simulink model "Analog_Solution"  (R2017a)
settings: Solver=FixedStepDiscrete  StartTime=0.0  StopTime=inf  FixedStep=Ts_main  RelTol=1e-3  EnableMultiTasking=on
InitFcn:
  | clc
  | eval('ContrPrm_v1_1')
model workspace (MAT data in the model file):
  JoyW_sat = 10
values from neighbouring files (symbols this model uses):
  Afilt_Winch = (Amatr_Winch-L_Winch*Cmatr_Winch)    [ContrPrm_v1_1.m]
  AOsat = 10    [ContrPrm_v1_1.m]
  Bfilt_Winch = [L_Winch Bmatr_Winch]    [ContrPrm_v1_1.m]
  Cfilt_Winch = eye(2)    [ContrPrm_v1_1.m]
  Dfilt_Winch = zeros(2)    [ContrPrm_v1_1.m]
  JoyS_gain = 5    [ContrPrm_v1_1.m]
  JoyS_ofst = -2.5    [ContrPrm_v1_1.m]
  JoyS_sat = 9.2    [ContrPrm_v1_1.m]
  JoyW_gain = -5    [ContrPrm_v1_1.m]
  JoyW_ofst = -2.5    [ContrPrm_v1_1.m]
  KspdWinch = 1    [ContrPrm_v1_1.m]
  NPotSpdEst = 3    [ContrPrm_v1_1.m]
  Pot_gain = PotMax/5    (= 0.08)    [ContrPrm_v1_1.m]
  Pot_max = PotMax    (= 0.4)    [ContrPrm_v1_1.m]
  Pot_min = 0    [ContrPrm_v1_1.m]
  Pot_ofst = -0.0558    [ContrPrm_v1_1.m]
  Ts_1ms = 1e-3    (= 0.001)    [ContrPrm_v1_1.m]
  Ts_1s = 1    [ContrPrm_v1_1.m]
  WinchDrumRad = 0.1    [ContrPrm_v1_1.m]
  WinchMotPosAIgain = WinchRevMax/WinchVoltMax*rev2rad    (= 76)    [ContrPrm_v1_1.m]
  WinchMotTorqueMax = 13    [ContrPrm_v1_1.m]
  WinchRefSpdSup = 15/WinchDrumRad    (= 150)    [ContrPrm_v1_1.m]
  WinchTravelMin_m = -2    [ContrPrm_v1_1.m]
  WinchVoltMax = 10    [ContrPrm_v1_1.m]
  x0_Winch = [0;0]    [ContrPrm_v1_1.m]
undefined symbols (not defined in the file or in its folder): datevec, JoyFiltDen, JoyFiltNum, PotPosFiltDen, PotPosFiltNum, WinchPosFiltDen, WinchPosFiltNum, WinchSpdEstFiltDen, WinchSpdEstFiltNum
libraries: slrtlib x10, xpcnilib x6, simulink x6, xpcseriallib x4, xpcwalltimelib x1
(part 2 of 3)

== system Analog_Solution/Startup/Initialize Spooling Position/FirstDirectionDone? ==
  SpoolingGrenze1 : Inport
  Constant1 : Constant
  Constant2 : Constant  Value=0
  Delay : Delay  DelayLength=1  InitialCondition=0
  Relational Operator : RelationalOperator  Operator=<=  OutDataTypeStr=boolean  RndMeth=Simplest
  Sum : Sum  Inputs=|++
  Switch1 : Switch  Criteria=u2 > Threshold
  Switch2 : Switch  Criteria=u2 > Threshold
  FirstDirectionDone : Outport
  wires:
  Switch1/1 -> Sum/1
  Delay/1 -> Sum/2
  SpoolingGrenze1/1 -> Switch1/2
  Constant2/1 -> Switch2/3, Switch1/3
  Sum/1 -> Delay/1, Relational Operator/2
  Constant1/1 -> Switch2/1, Relational Operator/1, Switch1/1
  Relational Operator/1 -> Switch2/2
  Switch2/1 -> FirstDirectionDone/1

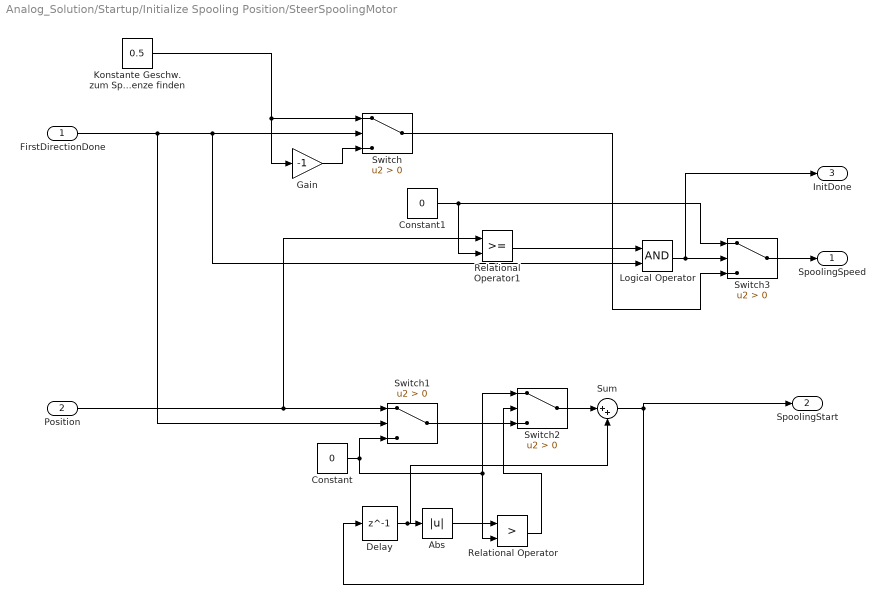
== system Analog_Solution/Startup/Initialize Spooling Position/SteerSpoolingMotor ==
  FirstDirectionDone : Inport
  Position : Inport  Port=2
  Abs : Abs
  Constant : Constant  Value=0
  Constant1 : Constant  Value=0
  Delay : Delay  DelayLength=1  InitialCondition=0
  Gain : Gain  Gain=-1
  Konstante Geschw. zum Spooling Grenze finden : Constant  Value=0.5
  Logical Operator : Logic  AllPortsSameDT=off  OutDataTypeStr=boolean
  Relational Operator : RelationalOperator  Operator=>  OutDataTypeStr=boolean  RndMeth=Simplest
  Relational Operator1 : RelationalOperator  OutDataTypeStr=boolean  RndMeth=Simplest
  Sum : Sum  Inputs=|++
  Switch{,1..3} (4 alike) : Switch  Criteria=u2 > Threshold
  SpoolingSpeed : Outport
  SpoolingStart : Outport  Port=2
  InitDone : Outport  Port=3
  wires:
  FirstDirectionDone/1 -> Switch1/2, Logical Operator/2, Switch/2
  Gain/1 -> Switch/3
  Konstante Geschw. zum Spooling Grenze finden/1 -> Gain/1, Switch/1
  Position/1 -> Relational Operator1/1, Switch1/1
  Sum/1 -> SpoolingStart/1, Delay/1
  Delay/1 -> Sum/2, Abs/1
  Relational Operator/1 -> Switch2/2
  Switch1/1 -> Switch2/3
  Abs/1 -> Relational Operator/1
  Switch2/1 -> Sum/1
  Constant/1 -> Switch2/1, Relational Operator/2, Switch1/3
  Logical Operator/1 -> InitDone/1, Switch3/2
  Switch/1 -> Switch3/3
  Relational Operator1/1 -> Logical Operator/1
  Constant1/1 -> Relational Operator1/2, Switch3/1
  Switch3/1 -> SpoolingSpeed/1

== system Analog_Solution/Winch_Conrtol/Joystick Regelung1/Joystick-Steuerung ==
  Joystick-Wert : Inport
  WinchSoll : Inport  Port=2
  Beschleunigung : Constant  Value=0.0006  SampleTime=0.001
  Gain : Gain  Gain=-1
  Relational Operator : RelationalOperator  OutDataTypeStr=boolean  RndMeth=Simplest
  Relational Operator1 : RelationalOperator  Operator=<  OutDataTypeStr=boolean  RndMeth=Simplest
  Sum : Sum  Inputs=|++
  Sum1 : Sum  Inputs=|++
  Switch : Switch  Criteria=u2 > Threshold
  Switch1 : Switch  Criteria=u2 > Threshold
  obere Grenze : Constant  SampleTime=0.001
  untere Grenze : Constant  Value=-1  SampleTime=0.001
  Out1 : Outport
  wires:
  Joystick-Wert/1 -> Relational Operator/1, Relational Operator1/1
  obere Grenze/1 -> Relational Operator/2
  Relational Operator/1 -> Switch/2
  untere Grenze/1 -> Relational Operator1/2
  Switch/1 -> Switch1/3
  Relational Operator1/1 -> Switch1/2
  Switch1/1 -> Out1/1
  WinchSoll/1 -> Sum1/2, Switch/3, Sum/2
  Beschleunigung/1 -> Gain/1, Sum/1
  Sum/1 -> Switch/1
  Gain/1 -> Sum1/1
  Sum1/1 -> Switch1/1

== system Analog_Solution/Winch_Conrtol/Joystick Regelung1/damper ==
  SollWert : Inport
  Beschleunigung : Constant  Value=0.00125  SampleTime=0.001
  Compare To Zero : simulink/Logic and Bit Operations/Compare To Zero  relop=>  OutDataTypeStr=boolean
  Compare To Zero1 : simulink/Logic and Bit Operations/Compare To Zero  relop=<  OutDataTypeStr=boolean
  Constant1 : Constant  Value=0  SampleTime=0.001
  Delay : Delay  DelayLength=1  InitialCondition=0
  Delay1 : Delay  DelayLength=1  InitialCondition=0
  Gain : Gain  Gain=-1
  Sum : Sum  Inputs=|+-
  Sum1 : Sum  Inputs=|++
  Switch : Switch  Criteria=u2 > Threshold
  Switch1 : Switch  Criteria=u2 > Threshold
  Out1 : Outport
  wires:
  Sum/1 -> Compare To Zero1/1, Compare To Zero/1
  Compare To Zero/1 -> Switch/2
  Constant1/1 -> Switch/3
  Compare To Zero1/1 -> Switch1/2
  Switch/1 -> Switch1/3
  Gain/1 -> Switch1/1
  SollWert/1 -> Sum/1
  Switch1/1 -> Sum1/1
  Sum1/1 -> Delay/1, Delay1/1, Out1/1
  Delay/1 -> Sum/2
  Delay1/1 -> Sum1/2
  Beschleunigung/1 -> Switch/1, Gain/1

== system Analog_Solution/Inputs/RS232_read/IMU_read/Data_Check_CRC ==
  ASCII_IMU_crc : Inport
  Demux : Demux  Outputs=[143 2]
  Embedded MATLAB Function : MATLAB Function  TreatAsAtomicUnit=on
  Enable : Outport
  wires:
  Demux/2 -> Embedded MATLAB Function/2(crc_in)
  Embedded MATLAB Function/1(CRC_valid) -> Enable/1
  ASCII_IMU_crc/1 -> Demux/1
  Demux/1 -> Embedded MATLAB Function/1(pBuffer)

== system Analog_Solution/Inputs/RS232_read/IMU_read/Data_validation ==
  IMU_data : Inport
  Enable : EnablePort
  IMU_data_valid : Outport
  wires:
  IMU_data/1 -> IMU_data_valid/1

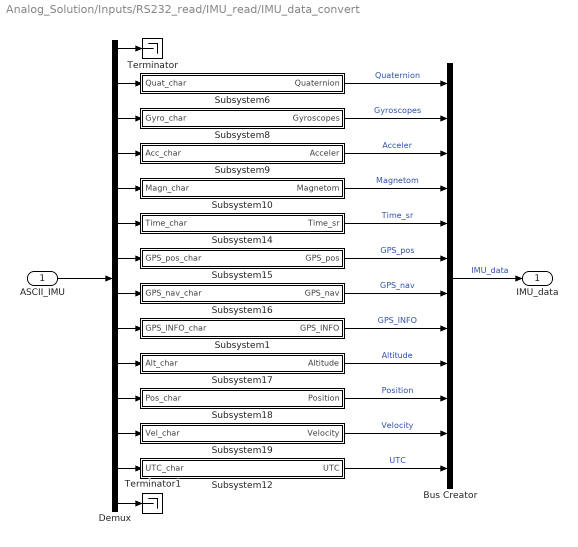
== system Analog_Solution/Inputs/RS232_read/IMU_read/IMU_data_convert ==
  ASCII_IMU : Inport
  Bus Creator : BusCreator  Inputs=12
  Demux : Demux  Outputs=[3 16 12 12 12 4 12 16 6 4 24 12 10 2]
  Subsystem1 : Subsystem
  Subsystem10 : Subsystem
  Subsystem12 : Subsystem
  Subsystem14 : Subsystem
  Subsystem15 : Subsystem
  Subsystem16 : Subsystem
  Subsystem17 : Subsystem
  Subsystem18 : Subsystem
  Subsystem19 : Subsystem
  Subsystem6 : Subsystem
  Subsystem8 : Subsystem
  Subsystem9 : Subsystem
  Terminator : Terminator
  Terminator1 : Terminator
  IMU_data : Outport
  wires:
  Bus Creator/1 -> IMU_data/1  "IMU_data"
  ASCII_IMU/1 -> Demux/1
  Demux/1 -> Terminator/1
  Demux/2 -> Subsystem6/1(Quat_char)
  Demux/3 -> Subsystem8/1(Gyro_char)
  Demux/4 -> Subsystem9/1(Acc_char)
  Demux/5 -> Subsystem10/1(Magn_char)
  Demux/6 -> Subsystem14/1(Time_char)
  Demux/14 -> Terminator1/1
  Subsystem6/1(Quaternion) -> Bus Creator/1  "Quaternion"
  Subsystem8/1(Gyroscopes) -> Bus Creator/2  "Gyroscopes"
  Subsystem9/1(Acceler) -> Bus Creator/3  "Acceler"
  Subsystem10/1(Magnetom) -> Bus Creator/4  "Magnetom"
  Subsystem14/1(Time_sr) -> Bus Creator/5  "Time_sr"
  Demux/7 -> Subsystem15/1(GPS_pos_char)
  Demux/8 -> Subsystem16/1(GPS_nav_char)
  Demux/9 -> Subsystem1/1(GPS_INFO_char)
  Demux/10 -> Subsystem17/1(Alt_char)
  Demux/11 -> Subsystem18/1(Pos_char)
  Demux/12 -> Subsystem19/1(Vel_char)
  Demux/13 -> Subsystem12/1(UTC_char)
  Subsystem15/1(GPS_pos) -> Bus Creator/6  "GPS_pos"
  Subsystem16/1(GPS_nav) -> Bus Creator/7  "GPS_nav"
  Subsystem1/1(GPS_INFO) -> Bus Creator/8  "GPS_INFO"
  Subsystem17/1(Altitude) -> Bus Creator/9  "Altitude"
  Subsystem18/1(Position) -> Bus Creator/10  "Position"
  Subsystem19/1(Velocity) -> Bus Creator/11  "Velocity"
  Subsystem12/1(UTC) -> Bus Creator/12  "UTC"

== system Analog_Solution/Inputs/RS232_read/IMU_read/IMU_data_convert/Subsystem1 ==
  GPS_INFO_char : Inport
  Bus Creator : BusCreator  Inputs=3
  Demux1 : Demux  Outputs=[4 1 1]
  Embedded MATLAB Function : MATLAB Function  TreatAsAtomicUnit=on
  Embedded MATLAB Function1 : MATLAB Function  TreatAsAtomicUnit=on
  Embedded MATLAB Function2 : MATLAB Function  TreatAsAtomicUnit=on
  GPS_INFO : Outport
  wires:
  GPS_INFO_char/1 -> Demux1/1
  Demux1/1 -> Embedded MATLAB Function/1(in)
  Embedded MATLAB Function/1(uint32_out) -> Bus Creator/1  "time"
  Demux1/2 -> Embedded MATLAB Function1/1(in)
  Demux1/3 -> Embedded MATLAB Function2/1(in)
  Embedded MATLAB Function1/1(uint8_out) -> Bus Creator/2  "GPSFlags"
  Embedded MATLAB Function2/1(uint8_out) -> Bus Creator/3  "NbSat"
  Bus Creator/1 -> GPS_INFO/1  "GPS_nav"

== system Analog_Solution/Inputs/RS232_read/IMU_read/IMU_data_convert/Subsystem10 ==
  Magn_char : Inport
  Bus Creator : BusCreator  Inputs=3
  Demux1 : Demux  Outputs=[4 4 4]
  Embedded MATLAB Function : MATLAB Function  TreatAsAtomicUnit=on
  Embedded MATLAB Function1 : MATLAB Function  TreatAsAtomicUnit=on
  Embedded MATLAB Function3 : MATLAB Function  TreatAsAtomicUnit=on
  Magnetom : Outport
  wires:
  Magn_char/1 -> Demux1/1
  Demux1/1 -> Embedded MATLAB Function/1(in)
  Demux1/2 -> Embedded MATLAB Function1/1(in)
  Demux1/3 -> Embedded MATLAB Function3/1(in)
  Embedded MATLAB Function/1(sing_out) -> Bus Creator/1  "Mx"
  Embedded MATLAB Function1/1(sing_out) -> Bus Creator/2  "My"
  Embedded MATLAB Function3/1(sing_out) -> Bus Creator/3  "Mz"
  Bus Creator/1 -> Magnetom/1  "Magnetom"

== system Analog_Solution/Inputs/RS232_read/IMU_read/IMU_data_convert/Subsystem12 ==
  UTC_char : Inport
  Bus Creator : BusCreator  Inputs=7
  Demux1 : Demux  Outputs=[1 1 1 1 1 1 4]
  Embedded MATLAB Function : MATLAB Function  TreatAsAtomicUnit=on
  Embedded MATLAB Function1 : MATLAB Function  TreatAsAtomicUnit=on
  Embedded MATLAB Function2 : MATLAB Function  TreatAsAtomicUnit=on
  Embedded MATLAB Function3 : MATLAB Function  TreatAsAtomicUnit=on
  Embedded MATLAB Function4 : MATLAB Function  TreatAsAtomicUnit=on
  Embedded MATLAB Function5 : MATLAB Function  TreatAsAtomicUnit=on
  Embedded MATLAB Function6 : MATLAB Function  TreatAsAtomicUnit=on
  UTC : Outport
  wires:
  UTC_char/1 -> Demux1/1
  Bus Creator/1 -> UTC/1  "UTC"
  Demux1/1 -> Embedded MATLAB Function/1(in)
  Demux1/2 -> Embedded MATLAB Function2/1(in)
  Demux1/3 -> Embedded MATLAB Function3/1(in)
  Demux1/4 -> Embedded MATLAB Function4/1(in)
  Demux1/5 -> Embedded MATLAB Function5/1(in)
  Demux1/6 -> Embedded MATLAB Function6/1(in)
  Demux1/7 -> Embedded MATLAB Function1/1(in)
  Embedded MATLAB Function/1(uint8_out) -> Bus Creator/1  "year"
  Embedded MATLAB Function2/1(uint8_out) -> Bus Creator/2  "month"
  Embedded MATLAB Function3/1(uint8_out) -> Bus Creator/3  "day"
  Embedded MATLAB Function4/1(uint8_out) -> Bus Creator/4  "hour"
  Embedded MATLAB Function5/1(uint8_out) -> Bus Creator/5  "min"
  Embedded MATLAB Function6/1(uint8_out) -> Bus Creator/6  "sec"
  Embedded MATLAB Function1/1(uint32_out) -> Bus Creator/7  "nanoseconds"

== system Analog_Solution/Inputs/RS232_read/IMU_read/IMU_data_convert/Subsystem14 ==
  Time_char : Inport
  Embedded MATLAB Function : MATLAB Function  TreatAsAtomicUnit=on
  Time_sr : Outport
  wires:
  Time_char/1 -> Embedded MATLAB Function/1(in)
  Embedded MATLAB Function/1(uint32_out) -> Time_sr/1  "Time_sr"

== system Analog_Solution/Inputs/RS232_read/IMU_read/IMU_data_convert/Subsystem15 ==
  GPS_pos_char : Inport
  Bus Creator : BusCreator  Inputs=3
  Demux1 : Demux  Outputs=[4 4 4]
  Embedded MATLAB Function1 : MATLAB Function  TreatAsAtomicUnit=on
  Embedded MATLAB Function2 : MATLAB Function  TreatAsAtomicUnit=on
  Embedded MATLAB Function3 : MATLAB Function  TreatAsAtomicUnit=on
  GPS_pos : Outport
  wires:
  GPS_pos_char/1 -> Demux1/1
  Bus Creator/1 -> GPS_pos/1  "GPS_pos"
  Embedded MATLAB Function2/1(int32_out) -> Bus Creator/3  "height"
  Embedded MATLAB Function1/1(int32_out) -> Bus Creator/2  "longitude"
  Embedded MATLAB Function3/1(int32_out) -> Bus Creator/1  "latitude"
  Demux1/3 -> Embedded MATLAB Function2/1(in)
  Demux1/2 -> Embedded MATLAB Function1/1(in)
  Demux1/1 -> Embedded MATLAB Function3/1(in)

== system Analog_Solution/Inputs/RS232_read/IMU_read/IMU_data_convert/Subsystem16 ==
  GPS_nav_char : Inport
  Bus Creator : BusCreator  Inputs=4
  Demux1 : Demux  Outputs=[4 4 4 4]
  Embedded MATLAB Function1 : MATLAB Function  TreatAsAtomicUnit=on
  Embedded MATLAB Function2 : MATLAB Function  TreatAsAtomicUnit=on
  Embedded MATLAB Function3 : MATLAB Function  TreatAsAtomicUnit=on
  Embedded MATLAB Function4 : MATLAB Function  TreatAsAtomicUnit=on
  GPS_nav : Outport
  wires:
  Demux1/1 -> Embedded MATLAB Function2/1(in)
  Demux1/2 -> Embedded MATLAB Function1/1(in)
  Demux1/3 -> Embedded MATLAB Function3/1(in)
  Embedded MATLAB Function2/1(int32_out) -> Bus Creator/1  "v_north"
  Embedded MATLAB Function1/1(int32_out) -> Bus Creator/2  "v_east"
  Embedded MATLAB Function3/1(int32_out) -> Bus Creator/3  "v_down"
  Bus Creator/1 -> GPS_nav/1  "GPS_nav"
  GPS_nav_char/1 -> Demux1/1
  Demux1/4 -> Embedded MATLAB Function4/1(in)
  Embedded MATLAB Function4/1(int32_out) -> Bus Creator/4  "heading"

== system Analog_Solution/Inputs/RS232_read/IMU_read/IMU_data_convert/Subsystem17 ==
  Alt_char : Inport
  Embedded MATLAB Function2 : MATLAB Function  TreatAsAtomicUnit=on
  Altitude : Outport
  wires:
  Alt_char/1 -> Embedded MATLAB Function2/1(in)
  Embedded MATLAB Function2/1(int32_out) -> Altitude/1  "Altitude"

== system Analog_Solution/Inputs/RS232_read/IMU_read/IMU_data_convert/Subsystem18 ==
  Pos_char : Inport
  Bus Creator : BusCreator  Inputs=3
  Demux1 : Demux  Outputs=[8 8 8]
  Embedded MATLAB Function : MATLAB Function  TreatAsAtomicUnit=on
  Embedded MATLAB Function1 : MATLAB Function  TreatAsAtomicUnit=on
  Embedded MATLAB Function2 : MATLAB Function  TreatAsAtomicUnit=on
  Position : Outport
  wires:
  Bus Creator/1 -> Position/1  "Position"
  Pos_char/1 -> Demux1/1
  Demux1/1 -> Embedded MATLAB Function/1(in)
  Demux1/2 -> Embedded MATLAB Function1/1(in)
  Demux1/3 -> Embedded MATLAB Function2/1(in)
  Embedded MATLAB Function2/1(double_out) -> Bus Creator/3  "height_filt"
  Embedded MATLAB Function1/1(double_out) -> Bus Creator/2  "long_filt"
  Embedded MATLAB Function/1(double_out) -> Bus Creator/1  "lat_filt"

== system Analog_Solution/Inputs/RS232_read/IMU_read/IMU_data_convert/Subsystem19 ==
  Vel_char : Inport
  Bus Creator : BusCreator  Inputs=3
  Demux1 : Demux  Outputs=[4 4 4]
  Embedded MATLAB Function : MATLAB Function  TreatAsAtomicUnit=on
  Embedded MATLAB Function1 : MATLAB Function  TreatAsAtomicUnit=on
  Embedded MATLAB Function3 : MATLAB Function  TreatAsAtomicUnit=on
  Velocity : Outport
  wires:
  Embedded MATLAB Function/1(sing_out) -> Bus Creator/1  "Vx"
  Embedded MATLAB Function1/1(sing_out) -> Bus Creator/2  "Vy"
  Embedded MATLAB Function3/1(sing_out) -> Bus Creator/3  "Vz"
  Demux1/3 -> Embedded MATLAB Function3/1(in)
  Demux1/2 -> Embedded MATLAB Function1/1(in)
  Demux1/1 -> Embedded MATLAB Function/1(in)
  Vel_char/1 -> Demux1/1
  Bus Creator/1 -> Velocity/1  "Velocity"

== system Analog_Solution/Inputs/RS232_read/IMU_read/IMU_data_convert/Subsystem6 ==
  Quat_char : Inport
  Bus Creator : BusCreator  Inputs=4
  Demux1 : Demux  Outputs=[4 4 4 4]
  Embedded MATLAB Function : MATLAB Function  TreatAsAtomicUnit=on
  Embedded MATLAB Function1 : MATLAB Function  TreatAsAtomicUnit=on
  Embedded MATLAB Function3 : MATLAB Function  TreatAsAtomicUnit=on
  Embedded MATLAB Function4 : MATLAB Function  TreatAsAtomicUnit=on
  Quaternion : Outport
  wires:
  Quat_char/1 -> Demux1/1
  Demux1/1 -> Embedded MATLAB Function/1(in)
  Demux1/2 -> Embedded MATLAB Function1/1(in)
  Demux1/3 -> Embedded MATLAB Function3/1(in)
  Demux1/4 -> Embedded MATLAB Function4/1(in)
  Embedded MATLAB Function/1(sing_out) -> Bus Creator/1  "q1"
  Embedded MATLAB Function1/1(sing_out) -> Bus Creator/2  "q2"
  Embedded MATLAB Function3/1(sing_out) -> Bus Creator/3  "q3"
  Embedded MATLAB Function4/1(sing_out) -> Bus Creator/4  "q4"
  Bus Creator/1 -> Quaternion/1  "Quaternion"

== system Analog_Solution/Inputs/RS232_read/IMU_read/IMU_data_convert/Subsystem8 ==
  Gyro_char : Inport
  Bus Creator : BusCreator  Inputs=3
  Demux1 : Demux  Outputs=[4 4 4]
  Embedded MATLAB Function : MATLAB Function  TreatAsAtomicUnit=on
  Embedded MATLAB Function1 : MATLAB Function  TreatAsAtomicUnit=on
  Embedded MATLAB Function3 : MATLAB Function  TreatAsAtomicUnit=on
  Gyroscopes : Outport
  wires:
  Gyro_char/1 -> Demux1/1
  Demux1/1 -> Embedded MATLAB Function/1(in)
  Demux1/2 -> Embedded MATLAB Function1/1(in)
  Demux1/3 -> Embedded MATLAB Function3/1(in)
  Embedded MATLAB Function/1(sing_out) -> Bus Creator/1  "Gx"
  Embedded MATLAB Function1/1(sing_out) -> Bus Creator/2  "Gy"
  Embedded MATLAB Function3/1(sing_out) -> Bus Creator/3  "Gz"
  Bus Creator/1 -> Gyroscopes/1  "Gyroscopes"

== system Analog_Solution/Inputs/RS232_read/IMU_read/IMU_data_convert/Subsystem9 ==
  Acc_char : Inport
  Bus Creator : BusCreator  Inputs=3
  Demux1 : Demux  Outputs=[4 4 4]
  Embedded MATLAB Function : MATLAB Function  TreatAsAtomicUnit=on
  Embedded MATLAB Function1 : MATLAB Function  TreatAsAtomicUnit=on
  Embedded MATLAB Function3 : MATLAB Function  TreatAsAtomicUnit=on
  Acceler : Outport
  wires:
  Bus Creator/1 -> Acceler/1  "Acceler"
  Embedded MATLAB Function3/1(sing_out) -> Bus Creator/3  "Az"
  Embedded MATLAB Function1/1(sing_out) -> Bus Creator/2  "Ay"
  Embedded MATLAB Function/1(sing_out) -> Bus Creator/1  "Ax"
  Demux1/3 -> Embedded MATLAB Function3/1(in)
  Demux1/2 -> Embedded MATLAB Function1/1(in)
  Demux1/1 -> Embedded MATLAB Function/1(in)
  Acc_char/1 -> Demux1/1

== matlab function Analog_Solution/Inputs/RS232_read/IMU_read/IMU_data_convert/Subsystem17/Embedded MATLAB Function2 ==
  data: in input; int32_out output
function int32_out=word2int32(in)%#eml

% in=double(in);
vec1=convert1word(in(1,1));
vec2=convert1word(in(2,1));
vec3=convert1word(in(3,1));
vec4=convert1word(in(4,1));

temp=[vec1 vec2 vec3 vec4];

int32_out=uint32_conv(temp(2:end))-temp(1)*2.147483648e9;

function vec=uint32_conv(in)
vec=0;
for ind=1:31;
    vec=vec+in(ind)*2^(31-ind);
end

function vec=convert1word(in)
vec=zeros(1,8);
ind=uint8(7);

while in>0;
    a=2^ind;
    if in>=a
        vec(1,8-ind)=1;
        in=in-a;
    else
        vec(1,8-ind)=0;
    end
    ind=ind-1;
end

== matlab function Analog_Solution/Inputs/RS232_read/IMU_read/IMU_data_convert/Subsystem18/Embedded MATLAB Function ==
  data: in input; double_out output
function double_out=word2double(in)%#eml

vec1=convert1word(in(1,1));
vec2=convert1word(in(2,1));
vec3=convert1word(in(3,1));
vec4=convert1word(in(4,1));
vec5=convert1word(in(5,1));
vec6=convert1word(in(6,1));
vec7=convert1word(in(7,1));
vec8=convert1word(in(8,1));

temp=[vec1 vec2 vec3 vec4 vec5 vec6 vec7 vec8];

exponent=exp_conv(temp(1,2:12));
signif=signif_conv(temp(1,13:end));
signum=sign_conv(temp(1,1));

if exponent==-1023 
    if signif==0;
        double_out=signum*0;
    else
        double_out=signum*2^-1022*signif;
    end
elseif exponent==1024
    if signif~=0;
        double_out=NaN;
    else
        double_out=signum*Inf;
    end
else
    double_out=signum*2^exponent*(1+signif);
end

function vec=convert1word(in)
vec=zeros(1,8);
ind=uint8(7);

while in>0;
    a=2^ind;
    if in>=a
        vec(1,8-ind)=1;
        in=in-a;
    else
        vec(1,8-ind)=0;
    end
    ind=ind-1;
end

function vec=sign_conv(in)
vec=(-1)^in;

function vec=exp_conv(in)
vec=0;
for ind=1:11;
    vec=vec+in(ind)*2^(11-ind);
end
vec=vec-1023;

function vec=signif_conv(in)
vec=0;
for ind=1:52;
    vec=vec+in(ind)*2^-ind;
end

== matlab function Analog_Solution/Inputs/RS232_read/IMU_read/IMU_data_convert/Subsystem18/Embedded MATLAB Function1 ==
  data: in input; double_out output
function double_out=word2double(in)%#eml

vec1=convert1word(in(1,1));
vec2=convert1word(in(2,1));
vec3=convert1word(in(3,1));
vec4=convert1word(in(4,1));
vec5=convert1word(in(5,1));
vec6=convert1word(in(6,1));
vec7=convert1word(in(7,1));
vec8=convert1word(in(8,1));

temp=[vec1 vec2 vec3 vec4 vec5 vec6 vec7 vec8];

exponent=exp_conv(temp(1,2:12));
signif=signif_conv(temp(1,13:end));
signum=sign_conv(temp(1,1));

if exponent==-1023 
    if signif==0;
        double_out=signum*0;
    else
        double_out=signum*2^-1022*signif;
    end
elseif exponent==1024
    if signif~=0;
        double_out=NaN;
    else
        double_out=signum*Inf;
    end
else
    double_out=signum*2^exponent*(1+signif);
end

function vec=convert1word(in)
vec=zeros(1,8);
ind=uint8(7);

while in>0;
    a=2^ind;
    if in>=a
        vec(1,8-ind)=1;
        in=in-a;
    else
        vec(1,8-ind)=0;
    end
    ind=ind-1;
end

function vec=sign_conv(in)
vec=(-1)^in;

function vec=exp_conv(in)
vec=0;
for ind=1:11;
    vec=vec+in(ind)*2^(11-ind);
end
vec=vec-1023;

function vec=signif_conv(in)
vec=0;
for ind=1:52;
    vec=vec+in(ind)*2^-ind;
end

== matlab function Analog_Solution/Inputs/RS232_read/GPS_read/Embedded MATLAB Function ==
  data: in input; GU_Lat output; GU_Lon output; GU_h output; Geo_GU_h output
function [GU_Lat,GU_Lon,GU_h,Geo_GU_h]=GPSread(in)%#codegen

% Message frame: $GPGGA,time(hhmmss),Latitude(ddmm.mmmm),Hemisphere(N or S),
% Longitude(dddmm.mmmm),Hemisphere(W or E),GPS quality,Number of satellites,
% Horizontal dilution of precision,Antenna height(-9999.9 to 99999.9 m),
% Geoidal height(-999.9 to 9999.9 m),null,null *hh 0d 0a

% Output: Latitude in deg, Longitude in deg, height in m, Geoidal height in m
% >0 for North and West

in_char=char(in);
in_double=double(in);
index_comma=find(in_char==',');

if in_char(1)=='$';
    
    Latitude=in_char(index_comma(2,1)+1:index_comma(3,1)-1);
    index_dot_Lat=find(Latitude=='.');
    GU_Lat=(in_double(index_comma(2,1)+index_dot_Lat(1,1)-4)-48)*1e1+...
        in_double(index_comma(2,1)+index_dot_Lat(1,1)-3)-48+...
        ((in_double(index_comma(2,1)+index_dot_Lat(1,1)-2)-48)*10+...
        in_double(index_comma(2,1)+index_dot_Lat(1,1)-1)-48+...
        (in_double(index_comma(2,1)+index_dot_Lat(1,1)+1)-48)*1e-1+...
        (in_double(index_comma(2,1)+index_dot_Lat(1,1)+2)-48)*1e-2+...
        (in_double(index_comma(2,1)+index_dot_Lat(1,1)+3)-48)*1e-3+...
        (in_double(index_comma(2,1)+index_dot_Lat(1,1)+4)-48)*1e-4)/60;
    Lat_sign=in_char(index_comma(3)+1);
    if Lat_sign=='S'
        GU_Lat=-1*GU_Lat;
    end
    
    Longitude=in_char(index_comma(4,1)+1:index_comma(5,1)-1);
    index_dot_Lon=find(Longitude=='.');
    GU_Lon=(in_double(index_comma(4,1)+index_dot_Lon(1,1)-5)-48)*1e2+...
        (in_double(index_comma(4,1)+index_dot_Lon(1,1)-4)-48)*1e1+...
        in_double(index_comma(4,1)+index_dot_Lon(1,1)-3)-48+...
        ((in_double(index_comma(4,1)+index_dot_Lon(1,1)-2)-48)*10+...
        in_double(index_comma(4,1)+index_dot_Lon(1,1)-1)-48+...
        (in_double(index_comma(4,1)+index_dot_Lon(1,1)+1)-48)*1e-1+...
        (in_double(index_comma(4,1)+index_dot_Lon(1,1)+2)-48)*1e-2+...
        (in_double(index_comma(4,1)+index_dot_Lon(1,1)+3)-48)*1e-3+...
        (in_double(index_comma(4,1)+index_dot_Lon(1,1)+4)-48)*1e-4)/60;
    Lon_sign=in_char(index_comma(5)+1);
    if Lon_sign=='W'
        GU_Lon=-1*GU_Lon;
    end
    
    Antenna_h=in_char(index_comma(9,1)+1:index_comma(10,1)-1);
    temp=find(Antenna_h=='.');
    index_dot_Ant_h=temp(1,1);
    GU_h=0;
    if in(index_comma(9,1)+1)==45;
        for ind=index_comma(9,1)+2:index_comma(9,1)+index_dot_Ant_h-1
            GU_h=GU_h-(in_double(ind)-48)*...
                10^(index_comma(9,1)+index_dot_Ant_h-1-ind);
        end
        GU_h=GU_h-0.1*(in_double(index_comma(9,1)+index_dot_Ant_h+1)-48);
    else
        for ind=index_comma(9,1)+1:index_comma(9,1)+index_dot_Ant_h-1
            GU_h=GU_h+(in_double(ind)-48)*...
                10^(index_comma(9,1)+index_dot_Ant_h-1-ind);
        end
        GU_h=GU_h+0.1*(in_double(index_comma(9,1)+index_dot_Ant_h+1)-48);
    end
    
    Geoidal_h=in_char(index_comma(11,1)+1:index_comma(12,1)-1);
    temp=find(Geoidal_h=='.');
    index_dot_Geo_h=temp(1,1);
    Geo_GU_h=0;
    if in(index_comma(11,1)+1)==45;
        for ind=index_comma(11,1)+2:index_comma(11,1)+index_dot_Geo_h-1
            Geo_GU_h=Geo_GU_h-(in_double(ind)-48)*...
                10^(index_comma(11,1)+index_dot_Geo_h-1-ind);
        end
        Geo_GU_h=Geo_GU_h-0.1*(in_double(index_comma(11,1)+index_dot_Geo_h+1)-48);
    else
        for ind=index_comma(11,1)+1:index_comma(11,1)+index_dot_Geo_h-1
            Geo_GU_h=Geo_GU_h+(in_double(ind)-48)*...
                10^(index_comma(11,1)+index_dot_Geo_h-1-ind);
        end
        Geo_GU_h=Geo_GU_h+0.1*(in_double(index_comma(11,1)+index_dot_Geo_h+1)-48);
    end
else
    GU_Lat=0;
    GU_Lon=0;
    GU_h=0;
    Geo_GU_h=0;
end

== matlab function Analog_Solution/Inputs/RS232_read/IMU_read/IMU_data_convert/Subsystem16/Embedded MATLAB Function2 ==
  data: in input; int32_out output
function int32_out=word2int32(in)%#eml

% in=double(in);
vec1=convert1word(in(1,1));
vec2=convert1word(in(2,1));
vec3=convert1word(in(3,1));
vec4=convert1word(in(4,1));

temp=[vec1 vec2 vec3 vec4];

int32_out=uint32_conv(temp(2:end))-temp(1)*2.147483648e9;

function vec=uint32_conv(in)
vec=0;
for ind=1:31;
    vec=vec+in(ind)*2^(31-ind);
end

function vec=convert1word(in)
vec=zeros(1,8);
ind=uint8(7);

while in>0;
    a=2^ind;
    if in>=a
        vec(1,8-ind)=1;
        in=in-a;
    else
        vec(1,8-ind)=0;
    end
    ind=ind-1;
end

== matlab function Analog_Solution/Inputs/RS232_read/IMU_read/IMU_data_convert/Subsystem16/Embedded MATLAB Function1 ==
  data: in input; int32_out output
function int32_out=word2int32(in)%#eml

% in=double(in);
vec1=convert1word(in(1,1));
vec2=convert1word(in(2,1));
vec3=convert1word(in(3,1));
vec4=convert1word(in(4,1));

temp=[vec1 vec2 vec3 vec4];

int32_out=uint32_conv(temp(2:end))-temp(1)*2.147483648e9;

function vec=uint32_conv(in)
vec=0;
for ind=1:31;
    vec=vec+in(ind)*2^(31-ind);
end

function vec=convert1word(in)
vec=zeros(1,8);
ind=uint8(7);

while in>0;
    a=2^ind;
    if in>=a
        vec(1,8-ind)=1;
        in=in-a;
    else
        vec(1,8-ind)=0;
    end
    ind=ind-1;
end

== matlab function Analog_Solution/Inputs/RS232_read/IMU_read/IMU_data_convert/Subsystem16/Embedded MATLAB Function3 ==
  data: in input; int32_out output
function int32_out=word2int32(in)%#eml

% in=double(in);
vec1=convert1word(in(1,1));
vec2=convert1word(in(2,1));
vec3=convert1word(in(3,1));
vec4=convert1word(in(4,1));

temp=[vec1 vec2 vec3 vec4];

int32_out=uint32_conv(temp(2:end))-temp(1)*2.147483648e9;

function vec=uint32_conv(in)
vec=0;
for ind=1:31;
    vec=vec+in(ind)*2^(31-ind);
end

function vec=convert1word(in)
vec=zeros(1,8);
ind=uint8(7);

while in>0;
    a=2^ind;
    if in>=a
        vec(1,8-ind)=1;
        in=in-a;
    else
        vec(1,8-ind)=0;
    end
    ind=ind-1;
end

== matlab function Analog_Solution/Inputs/RS232_read/IMU_read/IMU_data_convert/Subsystem6/Embedded MATLAB Function ==
  data: in input; sing_out output
function sing_out=word2single(in)%#eml

vec1=convert1word(in(1,1));
vec2=convert1word(in(2,1));
vec3=convert1word(in(3,1));
vec4=convert1word(in(4,1));

temp=[vec1 vec2 vec3 vec4];

if sum(temp(1,2:9))==8 && sum(temp(1,10:end))==0;
    sing_out=sign_conv(temp(1,1))*Inf;
elseif sum(temp(1,2:9))==8 && sum(temp(1,10:end))>0;
    sing_out=NaN;
else
    sing_out=sign_conv(temp(1,1))*2^exp_conv(temp(1,2:9))*(1+signif_conv(temp(1,10:end)));
end

function vec=convert1word(in)
vec=zeros(1,8);
ind=uint8(7);

while in>0;
    a=2^ind;
    if in>=a
        vec(1,8-ind)=1;
        in=in-a;
    else
        vec(1,8-ind)=0;
    end
    ind=ind-1;
end

function vec=sign_conv(in)
vec=(-1)^in;

function vec=exp_conv(in)
vec=0;
for ind=1:8;
    vec=vec+in(ind)*2^(8-ind);
end
vec=vec-127;

function vec=signif_conv(in)
vec=0;
for ind=1:23;
    vec=vec+in(ind)*2^-ind;
end

== matlab function Analog_Solution/Inputs/RS232_read/IMU_read/IMU_data_convert/Subsystem6/Embedded MATLAB Function1 ==
  data: in input; sing_out output
function sing_out=word2single(in)%#eml

vec1=convert1word(in(1,1));
vec2=convert1word(in(2,1));
vec3=convert1word(in(3,1));
vec4=convert1word(in(4,1));

temp=[vec1 vec2 vec3 vec4];

if sum(temp(1,2:9))==8 && sum(temp(1,10:end))==0;
    sing_out=sign_conv(temp(1,1))*Inf;
elseif sum(temp(1,2:9))==8 && sum(temp(1,10:end))>0;
    sing_out=NaN;
else
    sing_out=sign_conv(temp(1,1))*2^exp_conv(temp(1,2:9))*(1+signif_conv(temp(1,10:end)));
end

function vec=convert1word(in)
vec=zeros(1,8);
ind=uint8(7);

while in>0;
    a=2^ind;
    if in>=a
        vec(1,8-ind)=1;
        in=in-a;
    else
        vec(1,8-ind)=0;
    end
    ind=ind-1;
end

function vec=sign_conv(in)
vec=(-1)^in;

function vec=exp_conv(in)
vec=0;
for ind=1:8;
    vec=vec+in(ind)*2^(8-ind);
end
vec=vec-127;

function vec=signif_conv(in)
vec=0;
for ind=1:23;
    vec=vec+in(ind)*2^-ind;
end

== matlab function Analog_Solution/Inputs/RS232_read/IMU_read/IMU_data_convert/Subsystem6/Embedded MATLAB Function3 ==
  data: in input; sing_out output
function sing_out=word2single(in)%#eml

vec1=convert1word(in(1,1));
vec2=convert1word(in(2,1));
vec3=convert1word(in(3,1));
vec4=convert1word(in(4,1));

temp=[vec1 vec2 vec3 vec4];

if sum(temp(1,2:9))==8 && sum(temp(1,10:end))==0;
    sing_out=sign_conv(temp(1,1))*Inf;
elseif sum(temp(1,2:9))==8 && sum(temp(1,10:end))>0;
    sing_out=NaN;
else
    sing_out=sign_conv(temp(1,1))*2^exp_conv(temp(1,2:9))*(1+signif_conv(temp(1,10:end)));
end

function vec=convert1word(in)
vec=zeros(1,8);
ind=uint8(7);

while in>0;
    a=2^ind;
    if in>=a
        vec(1,8-ind)=1;
        in=in-a;
    else
        vec(1,8-ind)=0;
    end
    ind=ind-1;
end

function vec=sign_conv(in)
vec=(-1)^in;

function vec=exp_conv(in)
vec=0;
for ind=1:8;
    vec=vec+in(ind)*2^(8-ind);
end
vec=vec-127;

function vec=signif_conv(in)
vec=0;
for ind=1:23;
    vec=vec+in(ind)*2^-ind;
end

== matlab function Analog_Solution/Inputs/RS232_read/IMU_read/IMU_data_convert/Subsystem6/Embedded MATLAB Function4 ==
  data: in input; sing_out output
function sing_out=word2single(in)%#eml

vec1=convert1word(in(1,1));
vec2=convert1word(in(2,1));
vec3=convert1word(in(3,1));
vec4=convert1word(in(4,1));

temp=[vec1 vec2 vec3 vec4];

if sum(temp(1,2:9))==8 && sum(temp(1,10:end))==0;
    sing_out=sign_conv(temp(1,1))*Inf;
elseif sum(temp(1,2:9))==8 && sum(temp(1,10:end))>0;
    sing_out=NaN;
else
    sing_out=sign_conv(temp(1,1))*2^exp_conv(temp(1,2:9))*(1+signif_conv(temp(1,10:end)));
end

function vec=convert1word(in)
vec=zeros(1,8);
ind=uint8(7);

while in>0;
    a=2^ind;
    if in>=a
        vec(1,8-ind)=1;
        in=in-a;
    else
        vec(1,8-ind)=0;
    end
    ind=ind-1;
end

function vec=sign_conv(in)
vec=(-1)^in;

function vec=exp_conv(in)
vec=0;
for ind=1:8;
    vec=vec+in(ind)*2^(8-ind);
end
vec=vec-127;

function vec=signif_conv(in)
vec=0;
for ind=1:23;
    vec=vec+in(ind)*2^-ind;
end

== matlab function Analog_Solution/Inputs/RS232_read/IMU_read/IMU_data_convert/Subsystem8/Embedded MATLAB Function ==
  data: in input; sing_out output
function sing_out=word2single(in)%#eml

vec1=convert1word(in(1,1));
vec2=convert1word(in(2,1));
vec3=convert1word(in(3,1));
vec4=convert1word(in(4,1));

temp=[vec1 vec2 vec3 vec4];

if sum(temp(1,2:9))==8 && sum(temp(1,10:end))==0;
    sing_out=sign_conv(temp(1,1))*Inf;
elseif sum(temp(1,2:9))==8 && sum(temp(1,10:end))>0;
    sing_out=NaN;
else
    sing_out=sign_conv(temp(1,1))*2^exp_conv(temp(1,2:9))*(1+signif_conv(temp(1,10:end)));
end

function vec=convert1word(in)
vec=zeros(1,8);
ind=uint8(7);

while in>0;
    a=2^ind;
    if in>=a
        vec(1,8-ind)=1;
        in=in-a;
    else
        vec(1,8-ind)=0;
    end
    ind=ind-1;
end

function vec=sign_conv(in)
vec=(-1)^in;

function vec=exp_conv(in)
vec=0;
for ind=1:8;
    vec=vec+in(ind)*2^(8-ind);
end
vec=vec-127;

function vec=signif_conv(in)
vec=0;
for ind=1:23;
    vec=vec+in(ind)*2^-ind;
end

== matlab function Analog_Solution/Inputs/RS232_read/IMU_read/IMU_data_convert/Subsystem8/Embedded MATLAB Function1 ==
  data: in input; sing_out output
function sing_out=word2single(in)%#eml

vec1=convert1word(in(1,1));
vec2=convert1word(in(2,1));
vec3=convert1word(in(3,1));
vec4=convert1word(in(4,1));

temp=[vec1 vec2 vec3 vec4];

if sum(temp(1,2:9))==8 && sum(temp(1,10:end))==0;
    sing_out=sign_conv(temp(1,1))*Inf;
elseif sum(temp(1,2:9))==8 && sum(temp(1,10:end))>0;
    sing_out=NaN;
else
    sing_out=sign_conv(temp(1,1))*2^exp_conv(temp(1,2:9))*(1+signif_conv(temp(1,10:end)));
end

function vec=convert1word(in)
vec=zeros(1,8);
ind=uint8(7);

while in>0;
    a=2^ind;
    if in>=a
        vec(1,8-ind)=1;
        in=in-a;
    else
        vec(1,8-ind)=0;
    end
    ind=ind-1;
end

function vec=sign_conv(in)
vec=(-1)^in;

function vec=exp_conv(in)
vec=0;
for ind=1:8;
    vec=vec+in(ind)*2^(8-ind);
end
vec=vec-127;

function vec=signif_conv(in)
vec=0;
for ind=1:23;
    vec=vec+in(ind)*2^-ind;
end

== matlab function Analog_Solution/Inputs/RS232_read/IMU_read/IMU_data_convert/Subsystem8/Embedded MATLAB Function3 ==
  data: in input; sing_out output
function sing_out=word2single(in)%#eml

vec1=convert1word(in(1,1));
vec2=convert1word(in(2,1));
vec3=convert1word(in(3,1));
vec4=convert1word(in(4,1));

temp=[vec1 vec2 vec3 vec4];

if sum(temp(1,2:9))==8 && sum(temp(1,10:end))==0;
    sing_out=sign_conv(temp(1,1))*Inf;
elseif sum(temp(1,2:9))==8 && sum(temp(1,10:end))>0;
    sing_out=NaN;
else
    sing_out=sign_conv(temp(1,1))*2^exp_conv(temp(1,2:9))*(1+signif_conv(temp(1,10:end)));
end

function vec=convert1word(in)
vec=zeros(1,8);
ind=uint8(7);

while in>0;
    a=2^ind;
    if in>=a
        vec(1,8-ind)=1;
        in=in-a;
    else
        vec(1,8-ind)=0;
    end
    ind=ind-1;
end

function vec=sign_conv(in)
vec=(-1)^in;

function vec=exp_conv(in)
vec=0;
for ind=1:8;
    vec=vec+in(ind)*2^(8-ind);
end
vec=vec-127;

function vec=signif_conv(in)
vec=0;
for ind=1:23;
    vec=vec+in(ind)*2^-ind;
end

== matlab function Analog_Solution/Inputs/RS232_read/IMU_read/IMU_data_convert/Subsystem9/Embedded MATLAB Function ==
  data: in input; sing_out output
function sing_out=word2single(in)%#eml

vec1=convert1word(in(1,1));
vec2=convert1word(in(2,1));
vec3=convert1word(in(3,1));
vec4=convert1word(in(4,1));

temp=[vec1 vec2 vec3 vec4];

if sum(temp(1,2:9))==8 && sum(temp(1,10:end))==0;
    sing_out=sign_conv(temp(1,1))*Inf;
elseif sum(temp(1,2:9))==8 && sum(temp(1,10:end))>0;
    sing_out=NaN;
else
    sing_out=sign_conv(temp(1,1))*2^exp_conv(temp(1,2:9))*(1+signif_conv(temp(1,10:end)));
end

function vec=convert1word(in)
vec=zeros(1,8);
ind=uint8(7);

while in>0;
    a=2^ind;
    if in>=a
        vec(1,8-ind)=1;
        in=in-a;
    else
        vec(1,8-ind)=0;
    end
    ind=ind-1;
end

function vec=sign_conv(in)
vec=(-1)^in;

function vec=exp_conv(in)
vec=0;
for ind=1:8;
    vec=vec+in(ind)*2^(8-ind);
end
vec=vec-127;

function vec=signif_conv(in)
vec=0;
for ind=1:23;
    vec=vec+in(ind)*2^-ind;
end

== matlab function Analog_Solution/Inputs/RS232_read/IMU_read/IMU_data_convert/Subsystem9/Embedded MATLAB Function1 ==
  data: in input; sing_out output
function sing_out=word2single(in)%#eml

vec1=convert1word(in(1,1));
vec2=convert1word(in(2,1));
vec3=convert1word(in(3,1));
vec4=convert1word(in(4,1));

temp=[vec1 vec2 vec3 vec4];

if sum(temp(1,2:9))==8 && sum(temp(1,10:end))==0;
    sing_out=sign_conv(temp(1,1))*Inf;
elseif sum(temp(1,2:9))==8 && sum(temp(1,10:end))>0;
    sing_out=NaN;
else
    sing_out=sign_conv(temp(1,1))*2^exp_conv(temp(1,2:9))*(1+signif_conv(temp(1,10:end)));
end

function vec=convert1word(in)
vec=zeros(1,8);
ind=uint8(7);

while in>0;
    a=2^ind;
    if in>=a
        vec(1,8-ind)=1;
        in=in-a;
    else
        vec(1,8-ind)=0;
    end
    ind=ind-1;
end

function vec=sign_conv(in)
vec=(-1)^in;

function vec=exp_conv(in)
vec=0;
for ind=1:8;
    vec=vec+in(ind)*2^(8-ind);
end
vec=vec-127;

function vec=signif_conv(in)
vec=0;
for ind=1:23;
    vec=vec+in(ind)*2^-ind;
end

== matlab function Analog_Solution/Inputs/RS232_read/IMU_read/IMU_data_convert/Subsystem9/Embedded MATLAB Function3 ==
  data: in input; sing_out output
function sing_out=word2single(in)%#eml

vec1=convert1word(in(1,1));
vec2=convert1word(in(2,1));
vec3=convert1word(in(3,1));
vec4=convert1word(in(4,1));

temp=[vec1 vec2 vec3 vec4];

if sum(temp(1,2:9))==8 && sum(temp(1,10:end))==0;
    sing_out=sign_conv(temp(1,1))*Inf;
elseif sum(temp(1,2:9))==8 && sum(temp(1,10:end))>0;
    sing_out=NaN;
else
    sing_out=sign_conv(temp(1,1))*2^exp_conv(temp(1,2:9))*(1+signif_conv(temp(1,10:end)));
end

function vec=convert1word(in)
vec=zeros(1,8);
ind=uint8(7);

while in>0;
    a=2^ind;
    if in>=a
        vec(1,8-ind)=1;
        in=in-a;
    else
        vec(1,8-ind)=0;
    end
    ind=ind-1;
end

function vec=sign_conv(in)
vec=(-1)^in;

function vec=exp_conv(in)
vec=0;
for ind=1:8;
    vec=vec+in(ind)*2^(8-ind);
end
vec=vec-127;

function vec=signif_conv(in)
vec=0;
for ind=1:23;
    vec=vec+in(ind)*2^-ind;
end

== matlab function Analog_Solution/Inputs/RS232_read/IMU_read/IMU_data_convert/Subsystem10/Embedded MATLAB Function ==
  data: in input; sing_out output
function sing_out=word2single(in)%#eml

vec1=convert1word(in(1,1));
vec2=convert1word(in(2,1));
vec3=convert1word(in(3,1));
vec4=convert1word(in(4,1));

temp=[vec1 vec2 vec3 vec4];

if sum(temp(1,2:9))==8 && sum(temp(1,10:end))==0;
    sing_out=sign_conv(temp(1,1))*Inf;
elseif sum(temp(1,2:9))==8 && sum(temp(1,10:end))>0;
    sing_out=NaN;
else
    sing_out=sign_conv(temp(1,1))*2^exp_conv(temp(1,2:9))*(1+signif_conv(temp(1,10:end)));
end

function vec=convert1word(in)
vec=zeros(1,8);
ind=uint8(7);

while in>0;
    a=2^ind;
    if in>=a
        vec(1,8-ind)=1;
        in=in-a;
    else
        vec(1,8-ind)=0;
    end
    ind=ind-1;
end

function vec=sign_conv(in)
vec=(-1)^in;

function vec=exp_conv(in)
vec=0;
for ind=1:8;
    vec=vec+in(ind)*2^(8-ind);
end
vec=vec-127;

function vec=signif_conv(in)
vec=0;
for ind=1:23;
    vec=vec+in(ind)*2^-ind;
end

== matlab function Analog_Solution/Inputs/RS232_read/IMU_read/IMU_data_convert/Subsystem10/Embedded MATLAB Function1 ==
  data: in input; sing_out output
function sing_out=word2single(in)%#eml

vec1=convert1word(in(1,1));
vec2=convert1word(in(2,1));
vec3=convert1word(in(3,1));
vec4=convert1word(in(4,1));

temp=[vec1 vec2 vec3 vec4];

if sum(temp(1,2:9))==8 && sum(temp(1,10:end))==0;
    sing_out=sign_conv(temp(1,1))*Inf;
elseif sum(temp(1,2:9))==8 && sum(temp(1,10:end))>0;
    sing_out=NaN;
else
    sing_out=sign_conv(temp(1,1))*2^exp_conv(temp(1,2:9))*(1+signif_conv(temp(1,10:end)));
end

function vec=convert1word(in)
vec=zeros(1,8);
ind=uint8(7);

while in>0;
    a=2^ind;
    if in>=a
        vec(1,8-ind)=1;
        in=in-a;
    else
        vec(1,8-ind)=0;
    end
    ind=ind-1;
end

function vec=sign_conv(in)
vec=(-1)^in;

function vec=exp_conv(in)
vec=0;
for ind=1:8;
    vec=vec+in(ind)*2^(8-ind);
end
vec=vec-127;

function vec=signif_conv(in)
vec=0;
for ind=1:23;
    vec=vec+in(ind)*2^-ind;
end

== matlab function Analog_Solution/Inputs/RS232_read/IMU_read/IMU_data_convert/Subsystem10/Embedded MATLAB Function3 ==
  data: in input; sing_out output
function sing_out=word2single(in)%#eml

vec1=convert1word(in(1,1));
vec2=convert1word(in(2,1));
vec3=convert1word(in(3,1));
vec4=convert1word(in(4,1));

temp=[vec1 vec2 vec3 vec4];

if sum(temp(1,2:9))==8 && sum(temp(1,10:end))==0;
    sing_out=sign_conv(temp(1,1))*Inf;
elseif sum(temp(1,2:9))==8 && sum(temp(1,10:end))>0;
    sing_out=NaN;
else
    sing_out=sign_conv(temp(1,1))*2^exp_conv(temp(1,2:9))*(1+signif_conv(temp(1,10:end)));
end

function vec=convert1word(in)
vec=zeros(1,8);
ind=uint8(7);

while in>0;
    a=2^ind;
    if in>=a
        vec(1,8-ind)=1;
        in=in-a;
    else
        vec(1,8-ind)=0;
    end
    ind=ind-1;
end

function vec=sign_conv(in)
vec=(-1)^in;

function vec=exp_conv(in)
vec=0;
for ind=1:8;
    vec=vec+in(ind)*2^(8-ind);
end
vec=vec-127;

function vec=signif_conv(in)
vec=0;
for ind=1:23;
    vec=vec+in(ind)*2^-ind;
end

== matlab function Analog_Solution/Inputs/RS232_read/IMU_read/IMU_data_convert/Subsystem12/Embedded MATLAB Function1 ==
  data: in input; uint32_out output
function uint32_out=word2uint32(in)%#eml

vec1=convert1word(in(1,1));
vec2=convert1word(in(2,1));
vec3=convert1word(in(3,1));
vec4=convert1word(in(4,1));

temp=[vec1 vec2 vec3 vec4];

uint32_out=uint32_conv(temp);


function vec=uint32_conv(in)
vec=0;
for ind=1:32;
    vec=vec+in(ind)*2^(32-ind);
end

function vec=convert1word(in)
vec=zeros(1,8);
ind=uint8(7);

while in>0;
    a=2^ind;
    if in>=a
        vec(1,8-ind)=1;
        in=in-a;
    else
        vec(1,8-ind)=0;
    end
    ind=ind-1;
end

== matlab function Analog_Solution/Inputs/RS232_read/IMU_read/IMU_data_convert/Subsystem12/Embedded MATLAB Function2 ==
  data: in input; uint8_out output
function uint8_out=word2uint8(in)%#eml

vec1=convert1word(in(1,1));

temp=[vec1];

uint8_out=uint8_conv(temp);


function vec=uint8_conv(in)
vec=0;
for ind=1:8;
    vec=vec+in(ind)*2^(8-ind);
end

function vec=convert1word(in)
vec=zeros(1,8);
ind=uint8(7);

while in>0;
    a=2^ind;
    if in>=a
        vec(1,8-ind)=1;
        in=in-a;
    else
        vec(1,8-ind)=0;
    end
    ind=ind-1;
end

== matlab function Analog_Solution/Inputs/RS232_read/IMU_read/IMU_data_convert/Subsystem12/Embedded MATLAB Function3 ==
  data: in input; uint8_out output
function uint8_out=word2uint8(in)%#eml

vec1=convert1word(in(1,1));

temp=[vec1];

uint8_out=uint8_conv(temp);


function vec=uint8_conv(in)
vec=0;
for ind=1:8;
    vec=vec+in(ind)*2^(8-ind);
end

function vec=convert1word(in)
vec=zeros(1,8);
ind=uint8(7);

while in>0;
    a=2^ind;
    if in>=a
        vec(1,8-ind)=1;
        in=in-a;
    else
        vec(1,8-ind)=0;
    end
    ind=ind-1;
end

== matlab function Analog_Solution/Inputs/RS232_read/IMU_read/IMU_data_convert/Subsystem12/Embedded MATLAB Function ==
  data: in input; uint8_out output
function uint8_out=word2uint8(in)%#eml

vec1=convert1word(in(1,1));

temp=[vec1];

uint8_out=uint8_conv(temp);


function vec=uint8_conv(in)
vec=0;
for ind=1:8;
    vec=vec+in(ind)*2^(8-ind);
end

function vec=convert1word(in)
vec=zeros(1,8);
ind=uint8(7);

while in>0;
    a=2^ind;
    if in>=a
        vec(1,8-ind)=1;
        in=in-a;
    else
        vec(1,8-ind)=0;
    end
    ind=ind-1;
end

== matlab function Analog_Solution/Inputs/RS232_read/IMU_read/IMU_data_convert/Subsystem12/Embedded MATLAB Function4 ==
  data: in input; uint8_out output
function uint8_out=word2uint8(in)%#eml

vec1=convert1word(in(1,1));

temp=[vec1];

uint8_out=uint8_conv(temp);


function vec=uint8_conv(in)
vec=0;
for ind=1:8;
    vec=vec+in(ind)*2^(8-ind);
end

function vec=convert1word(in)
vec=zeros(1,8);
ind=uint8(7);

while in>0;
    a=2^ind;
    if in>=a
        vec(1,8-ind)=1;
        in=in-a;
    else
        vec(1,8-ind)=0;
    end
    ind=ind-1;
end

== matlab function Analog_Solution/Inputs/RS232_read/IMU_read/IMU_data_convert/Subsystem12/Embedded MATLAB Function5 ==
  data: in input; uint8_out output
function uint8_out=word2uint8(in)%#eml

vec1=convert1word(in(1,1));

temp=[vec1];

uint8_out=uint8_conv(temp);


function vec=uint8_conv(in)
vec=0;
for ind=1:8;
    vec=vec+in(ind)*2^(8-ind);
end

function vec=convert1word(in)
vec=zeros(1,8);
ind=uint8(7);

while in>0;
    a=2^ind;
    if in>=a
        vec(1,8-ind)=1;
        in=in-a;
    else
        vec(1,8-ind)=0;
    end
    ind=ind-1;
end

== matlab function Analog_Solution/Inputs/RS232_read/IMU_read/IMU_data_convert/Subsystem12/Embedded MATLAB Function6 ==
  data: in input; uint8_out output
function uint8_out=word2uint8(in)%#eml

vec1=convert1word(in(1,1));

temp=[vec1];

uint8_out=uint8_conv(temp);


function vec=uint8_conv(in)
vec=0;
for ind=1:8;
    vec=vec+in(ind)*2^(8-ind);
end

function vec=convert1word(in)
vec=zeros(1,8);
ind=uint8(7);

while in>0;
    a=2^ind;
    if in>=a
        vec(1,8-ind)=1;
        in=in-a;
    else
        vec(1,8-ind)=0;
    end
    ind=ind-1;
end

== matlab function Analog_Solution/Inputs/RS232_read/IMU_read/IMU_data_convert/Subsystem1/Embedded MATLAB Function ==
  data: in input; uint32_out output
function uint32_out=word2uint32(in)%#eml

vec1=convert1word(in(1,1));
vec2=convert1word(in(2,1));
vec3=convert1word(in(3,1));
vec4=convert1word(in(4,1));

temp=[vec1 vec2 vec3 vec4];

uint32_out=uint32_conv(temp);


function vec=uint32_conv(in)
vec=0;
for ind=1:32;
    vec=vec+in(ind)*2^(32-ind);
end

function vec=convert1word(in)
vec=zeros(1,8);
ind=uint8(7);

while in>0;
    a=2^ind;
    if in>=a
        vec(1,8-ind)=1;
        in=in-a;
    else
        vec(1,8-ind)=0;
    end
    ind=ind-1;
end

== matlab function Analog_Solution/Inputs/RS232_read/IMU_read/IMU_data_convert/Subsystem1/Embedded MATLAB Function1 ==
  data: in input; uint8_out output
function uint8_out=word2uint8(in)%#eml

vec1=convert1word(in(1,1));

temp=[vec1];

uint8_out=uint8_conv(temp);


function vec=uint8_conv(in)
vec=0;
for ind=1:8;
    vec=vec+in(ind)*2^(8-ind);
end

function vec=convert1word(in)
vec=zeros(1,8);
ind=uint8(7);

while in>0;
    a=2^ind;
    if in>=a
        vec(1,8-ind)=1;
        in=in-a;
    else
        vec(1,8-ind)=0;
    end
    ind=ind-1;
end

== matlab function Analog_Solution/Inputs/RS232_read/IMU_read/IMU_data_convert/Subsystem14/Embedded MATLAB Function ==
  data: in input; uint32_out output
function uint32_out=word2uint32(in)%#eml

vec1=convert1word(in(1,1));
vec2=convert1word(in(2,1));
vec3=convert1word(in(3,1));
vec4=convert1word(in(4,1));

temp=[vec1 vec2 vec3 vec4];

uint32_out=uint32_conv(temp);


function vec=uint32_conv(in)
vec=0;
for ind=1:32;
    vec=vec+in(ind)*2^(32-ind);
end

function vec=convert1word(in)
vec=zeros(1,8);
ind=uint8(7);

while in>0;
    a=2^ind;
    if in>=a
        vec(1,8-ind)=1;
        in=in-a;
    else
        vec(1,8-ind)=0;
    end
    ind=ind-1;
end

== matlab function Analog_Solution/Inputs/RS232_read/IMU_read/IMU_data_convert/Subsystem15/Embedded MATLAB Function3 ==
  data: in input; int32_out output
function int32_out=word2int32(in)%#eml

% in=double(in);
vec1=convert1word(in(1,1));
vec2=convert1word(in(2,1));
vec3=convert1word(in(3,1));
vec4=convert1word(in(4,1));

temp=[vec1 vec2 vec3 vec4];

int32_out=uint32_conv(temp(2:end))-temp(1)*2.147483648e9;

function vec=uint32_conv(in)
vec=0;
for ind=1:31;
    vec=vec+in(ind)*2^(31-ind);
end

function vec=convert1word(in)
vec=zeros(1,8);
ind=uint8(7);

while in>0;
    a=2^ind;
    if in>=a
        vec(1,8-ind)=1;
        in=in-a;
    else
        vec(1,8-ind)=0;
    end
    ind=ind-1;
end

== matlab function Analog_Solution/Inputs/RS232_read/IMU_read/IMU_data_convert/Subsystem15/Embedded MATLAB Function1 ==
  data: in input; int32_out output
function int32_out=word2int32(in)%#eml

% in=double(in);
vec1=convert1word(in(1,1));
vec2=convert1word(in(2,1));
vec3=convert1word(in(3,1));
vec4=convert1word(in(4,1));

temp=[vec1 vec2 vec3 vec4];

int32_out=uint32_conv(temp(2:end))-temp(1)*2.147483648e9;

function vec=uint32_conv(in)
vec=0;
for ind=1:31;
    vec=vec+in(ind)*2^(31-ind);
end

function vec=convert1word(in)
vec=zeros(1,8);
ind=uint8(7);

while in>0;
    a=2^ind;
    if in>=a
        vec(1,8-ind)=1;
        in=in-a;
    else
        vec(1,8-ind)=0;
    end
    ind=ind-1;
end

== matlab function Analog_Solution/Inputs/RS232_read/IMU_read/IMU_data_convert/Subsystem15/Embedded MATLAB Function2 ==
  data: in input; int32_out output
function int32_out=word2int32(in)%#eml

% in=double(in);
vec1=convert1word(in(1,1));
vec2=convert1word(in(2,1));
vec3=convert1word(in(3,1));
vec4=convert1word(in(4,1));

temp=[vec1 vec2 vec3 vec4];

int32_out=uint32_conv(temp(2:end))-temp(1)*2.147483648e9;

function vec=uint32_conv(in)
vec=0;
for ind=1:31;
    vec=vec+in(ind)*2^(31-ind);
end

function vec=convert1word(in)
vec=zeros(1,8);
ind=uint8(7);

while in>0;
    a=2^ind;
    if in>=a
        vec(1,8-ind)=1;
        in=in-a;
    else
        vec(1,8-ind)=0;
    end
    ind=ind-1;
end

== matlab function Analog_Solution/Inputs/RS232_read/IMU_read/IMU_data_convert/Subsystem16/Embedded MATLAB Function4 ==
  data: in input; int32_out output
function int32_out=word2int32(in)%#eml

% in=double(in);
vec1=convert1word(in(1,1));
vec2=convert1word(in(2,1));
vec3=convert1word(in(3,1));
vec4=convert1word(in(4,1));

temp=[vec1 vec2 vec3 vec4];

int32_out=uint32_conv(temp(2:end))-temp(1)*2.147483648e9;

function vec=uint32_conv(in)
vec=0;
for ind=1:31;
    vec=vec+in(ind)*2^(31-ind);
end

function vec=convert1word(in)
vec=zeros(1,8);
ind=uint8(7);

while in>0;
    a=2^ind;
    if in>=a
        vec(1,8-ind)=1;
        in=in-a;
    else
        vec(1,8-ind)=0;
    end
    ind=ind-1;
end
